simulink model "flattening_2_test"  (Simulink 9.0)
settings: Solver=FixedStepAuto  StartTime=0.0  StopTime=10.0  FixedStep=1.000000  RelTol=1e-3  EnableMultiTasking=on
settings Model: SuppressorTable=22 serialization::archive 11 0 6 0 0 0 0 0  Creator=arnaud  LastModifiedBy=hbourbou
settings DataIOCC: LimitDataPoints=on  SignalLoggingSaveFormat=ModelDataLogs
settings OptimizationCC: ExpressionDepthLimit=2147483647
settings DebuggingCC: SolverPrmCheckMsg=warning  FcnCallInpInsideContextMsg=warning  StateNameClashWarn=warning  StrictBusMsg=Warning
settings GRTTargetCC: CombineOutputUpdateFcns=off  GRTInterface=on

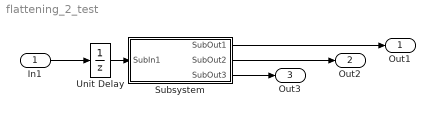
== system flattening_2_test ==
  In1 : Inport
  Subsystem : Subsystem
  Unit Delay : UnitDelay
  Out1 : Outport
  Out2 : Outport  Port=2
  Out3 : Outport  Port=3
  wires:
  Subsystem/1(SubOut1) -> Out1/1
  Subsystem/2(SubOut2) -> Out2/1
  Unit Delay/1 -> Subsystem/1(SubIn1)
  In1/1 -> Unit Delay/1
  Subsystem/3(SubOut3) -> Out3/1

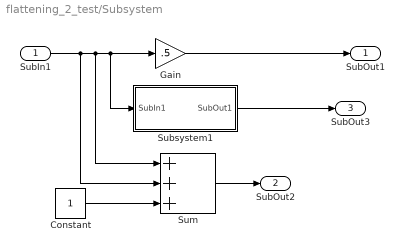
== system flattening_2_test/Subsystem ==
  SubIn1 : Inport
  Constant : Constant
  Gain : Gain  Gain=.5
  Subsystem1 : Subsystem
  Sum : Sum  Inputs=+++
  SubOut1 : Outport
  SubOut2 : Outport  Port=2
  SubOut3 : Outport  Port=3
  wires:
  SubIn1/1 -> Subsystem1/1(SubIn1), Gain/1, Sum/1, Sum/2
  Gain/1 -> SubOut1/1
  Sum/1 -> SubOut2/1
  Constant/1 -> Sum/3
  Subsystem1/1(SubOut1) -> SubOut3/1

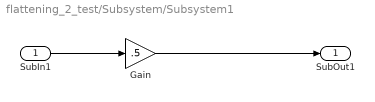
== system flattening_2_test/Subsystem/Subsystem1 ==
  SubIn1 : Inport
  Gain : Gain  Gain=.5
  SubOut1 : Outport
  wires:
  Gain/1 -> SubOut1/1
  SubIn1/1 -> Gain/1
